simulink model "windEmulatorStep4"  (R2025b)
settings: Solver=ode4  StartTime=0.0  StopTime=inf  FixedStep=Ts  RelTol=1e-3
values from neighbouring files (symbols this model uses):
  A = 1.0    (= 1)    [initStep4.m]
  absEncoderCountsToRad = 1/2^20*2*pi    (= 5.99211245268e-06)    [initStep4.m]
  acs800CtrlStruct =     [windEmulatorBusDefs.mat]
  acs800DcBusVoltsScaling = 1    [initStep4.m]
  acs800FreqScaling = 1/100    (= 0.01)    [initStep4.m]
  acs800PowerScaling = Gen_PowerScaling    (= 14.9109)    [initStep4.m]
  acs800SignalStruct =     [windEmulatorBusDefs.mat]
  acs800SpeedNomEng = 1500    [initStep4.m]
  acs800SpeedNomFb = 20000    [initStep4.m]
  acs800SpeedScaling = 1500/20000    (= 0.075)    [initStep4.m]
  acs800TempScaling = 1/10    (= 0.1)    [initStep4.m]
  acs800TorqueNomEng = 100    [initStep4.m]
  acs800TorqueNomFb = 10000    [initStep4.m]
  acs800TorqueScaling = acs800TorqueRating/10000    (= 0.008035933)    [initStep4.m]
  acs880CtrlStruct =     [windEmulatorBusDefs.mat]
  acs880FreqScaling = 60/20000    (= 0.003)    [initStep4.m]
  acs880MotorCurrentScaling = 100/10000    (= 0.01)    [initStep4.m]
  acs880MotorVoltsScaling = 1    [initStep4.m]
  acs880PowerScaling = 100*hp2W/10000    (= 7.457)    [initStep4.m]
  acs880RatedTorque = 80.494    [initStep4.m]
  acs880RateLimFalling = -10000    [initStep4.m]
  acs880RateLimRising = 10000    [initStep4.m]
  acs880SetpointLimLower = -0.975*acs880RatedTorque    (= -78.48165)    [initStep4.m]
  acs880SetpointLimUpper = 0.975*acs880RatedTorque    (= 78.48165)    [initStep4.m]
  acs880SignalStruct =     [windEmulatorBusDefs.mat]
  acs880SpeedPILimLo = -0.975*acs880RatedTorque    (= -78.48165)    [initStep4.m]
  acs880SpeedPILimUp = 0.975*acs880RatedTorque    (= 78.48165)    [initStep4.m]
  acs880SpeedScaling = 2000/20000    (= 0.1)    [initStep4.m]
  acs880TorqueFieldbusScale = 10000    [initStep4.m]
  acs880TorqueScaling = acs880RatedTorque/acs880TorqueFieldbusScale    (= 0.0080494)    [initStep4.m]
  acs880TorqueSetpointScaling = 100    [initStep4.m]
  bar2pa = 1e5    (= 100000)    [initStep4.m]
  belowMinPGain = 1/200    (= 0.005)    [initStep4.m]
  ctrlModeTorque = logical(true)    [init.m]    (also in initStep1.m; initStep2.m; initStep3.m; initStep4.m)
  ctrlSignal1 = squeeze(hptoSignalsData.Values.ctrlSignal1.Data)    [postProcessingStep2.m]
  ctrlSignal2 = squeeze(hptoSignalsData.Values.ctrlSignal2.Data)    [postProcessingStep2.m]
  deadBandController = boolean(false)    [initStep4.m]
  deadbandTorqueSlewRate = 300    [initStep4.m]
  Dm_max = 40    [initStep4.m]
  EffMechMax = 0.93    [initStep4.m]
  EffMechMin = 0.79    [initStep4.m]
  excForce_N = squeeze(hptoCtrlData.Values.excForce_N.Data)    [postProcessingStep2.m]
  expCtrlStruct =     [windEmulatorBusDefs.mat]
  FactorEff = psi2pa*cc2m3*(1/rev2rad)    (= 0.00109733470463)    [initStep4.m]
  fromFileSpeedSlewRate = 250    [initStep4.m]
  fromFileTorqueSlewRate = 25    [initStep4.m]
  futekTorqueScale = -1/(2^31)*10/5*100    (= -9.31322574615e-08)    [initStep4.m]
  genMaxTorque = 0.8*ratedTorque    (= 64.3952)    [initStep3.m]    (also in initStep4.m = 78.48165)
  genTorqueCmd_Nm = squeeze(hptoSignalsData.Values.genTorqueCmd_Nm.Data)    [postProcessingStep2.m]
  hbmCtScale = 1/1.5    (= 0.666666666667)    [initStep4.m]
  hbmPowerStruct =     [windEmulatorBusDefs.mat]
  hptoCtrlStruct =     [windEmulatorBusDefs.mat]
  hptoSignalStruct =     [windEmulatorBusDefs.mat]
  invPowerStruct =     [windEmulatorBusDefs.mat]
  lpm2m3ps = 1/m3ps2lpm    (= 1.66666666667e-05)    [initStep4.m]
  minPressureRef_psi = 1000    [initStep4.m]
  minTorqueRef_Nm = (minPressureRef_psi*psi2pa)*(Dm_max*cc2m3*(1/rev2rad))    (= 43.8933881851)    [initStep4.m]
  motorSpeed_rpm = squeeze(acs880SignalsData.Values.motorSpeed_rpm.Data)    [postProcessingStep2.m]
  nPreDrop = 2900    [initStep4.m]
  nPreDropMin = 725    [initStep4.m]
  psi2bar = 1/bar2psi    (= 0.0689475729318)    [initStep4.m]
  radps2rpm = 60/(2*pi)    (= 9.54929658551)    [initStep2.m]    (also in initStep4.m)
  rpm2radps = 2*pi/60    (= 0.10471975512)    [initStep4.m]
  runCounter = squeeze(hptoCtrlData.Values.runCounter.Data)    [postProcessingStep2.m]
  shaftSignalStruct =     [windEmulatorBusDefs.mat]
  sidCtrlStruct =     [windEmulatorBusDefs.mat]
  sidDataCaseCounter = sidData.experimentData.count    [initStep4.m]
  sidDataSpeed_rpm = sidData.experimentData.wShaft_rpm    [initStep4.m]
  sidDataTorque_Nm = sidData.experimentData.torqueShaft_Nm    [initStep4.m]
  sidInfoStruct =     [windEmulatorBusDefs.mat]
  T = 4    [initStep4.m]
  targetOmega = 2000/60*2*pi    (= 209.439510239)    [initStep2.m]    (also in initStep3.m; initStep4.m)
  time = hptoCtrlData.Values.runCounter.Time    [postProcessingStep2.m]
  TorqueLoadMax = 75    [initStep4.m]
  Ts = 1/250    (= 0.004)    [initStep4.m]
undefined symbols (not defined in the file or in its folder): absEncoderCounts, absEncoderPosition_rad, absEncoderSpeed_rpm, absEncoderStatus1, absEncoderStatus2, absEncoderTurns, acs800Torque_Nm, acs800TorqueSetpoint_Nm, acs880SpeedSetpoint_rpm, acs880Torque_Nm, ctrlWord, dcBusVoltage_V, DiscIntNeverNeededParam, excShaftSpeed_rpm, excShaftTorque_Nm, expType, expTypeEnum, frequency_Hz, fromFileCaseCounter, genPumpFlow_lpm, genShaftSpeed_rpm, genSpeedActual, hmOutputShafTorque_Nm, motorCurrent_A, motorTorque_Nm, motorVoltage_V, pressure_bar, PressureControl, ramp, resetHilIntegrator, resetSidIntegrator, runHil, runSid, shaftPower_W, sidType, sidTypeEnum, SpeedControl, speedCtrlReset, speedRef_rpm, state, statusWord, stepCounter, temperature, torqueActual_Nm, TorqueInputControl, torqueSetpoint_Nm, torqueSetpoint_percent
libraries: slrealtimeethercatlib x118, fl_lib x26, nesl_utility x17, slrealtimeloglib x13, sh_lib x9, dspstat3 x5, simulink_extras x4, slpidlib x3, cstblocks x3, dspindex x3, simulink x2
(part 3 of 5)

== system windEmulatorStep4/fileAndUI/expCtrlSignalsUI ==
  expCtrlSignals : Inport  OutDataTypeStr=Bus: expCtrlBus
  Bus Selector : BusSelector  OutputSignals=expType,runHil,runSid,resetHilIntegrator,resetSidIntegrator,time,ramp,runCounter,stepCounter
  Constant : Constant  Value=true
  Terminator{,1..8} (9 alike) : Terminator
  expType : Bias  SaturateOnIntegerOverflow=off
  ramp : Gain
  resetHilIntegrator : Logic  IconShape=distinctive  AllPortsSameDT=off  OutDataTypeStr=boolean
  resetSidIntegrator : Logic  IconShape=distinctive  AllPortsSameDT=off  OutDataTypeStr=boolean
  runCounter : Bias  SaturateOnIntegerOverflow=off
  runHil : Logic  IconShape=distinctive  AllPortsSameDT=off  OutDataTypeStr=boolean
  runSid : Logic  IconShape=distinctive  AllPortsSameDT=off  OutDataTypeStr=boolean
  stepCounter : Bias  SaturateOnIntegerOverflow=off
  time : Gain
  wires:
  expCtrlSignals/1 -> Bus Selector/1
  Bus Selector/1 -> expType/1  "<expType>"
  expType/1 -> Terminator/1
  Bus Selector/2 -> runHil/2  "<runHil>"
  Constant/1 -> resetSidIntegrator/1, resetHilIntegrator/1, runSid/1, runHil/1
  runHil/1 -> Terminator1/1
  Bus Selector/3 -> runSid/2  "<runSid>"
  runSid/1 -> Terminator2/1
  Bus Selector/4 -> resetHilIntegrator/2  "<resetHilIntegrator>"
  resetHilIntegrator/1 -> Terminator3/1
  Bus Selector/5 -> resetSidIntegrator/2  "<resetSidIntegrator>"
  resetSidIntegrator/1 -> Terminator4/1
  Bus Selector/8 -> runCounter/1  "<runCounter>"
  runCounter/1 -> Terminator5/1
  Bus Selector/6 -> time/1  "<time>"
  time/1 -> Terminator6/1
  Bus Selector/7 -> ramp/1  "<ramp>"
  ramp/1 -> Terminator7/1
  Bus Selector/9 -> stepCounter/1  "<stepCounter>"
  stepCounter/1 -> Terminator8/1

== system windEmulatorStep4/fileAndUI/hptoCtrlSignalsUI ==
  hptoCtrlSignals : Inport  OutDataTypeStr=Bus: hptoCtrlBus
  Bus Selector : BusSelector  OutputSignals=speedRef_rpm,excForce_N,genSpeedActual,speedCtrlReset
  Terminator{,1,4,6} (4 alike) : Terminator
  excForce_N : Gain
  genSpeedActual : Gain
  speedCtrlReset : Gain
  speedRef_rpm : Gain
  wires:
  hptoCtrlSignals/1 -> Bus Selector/1
  Bus Selector/1 -> speedRef_rpm/1  "<speedRef_rpm>"
  speedRef_rpm/1 -> Terminator/1
  Bus Selector/2 -> excForce_N/1  "<excForce_N>"
  excForce_N/1 -> Terminator1/1
  Bus Selector/3 -> genSpeedActual/1  "<genSpeedActual>"
  genSpeedActual/1 -> Terminator4/1
  Bus Selector/4 -> speedCtrlReset/1  "<speedCtrlReset>"
  speedCtrlReset/1 -> Terminator6/1

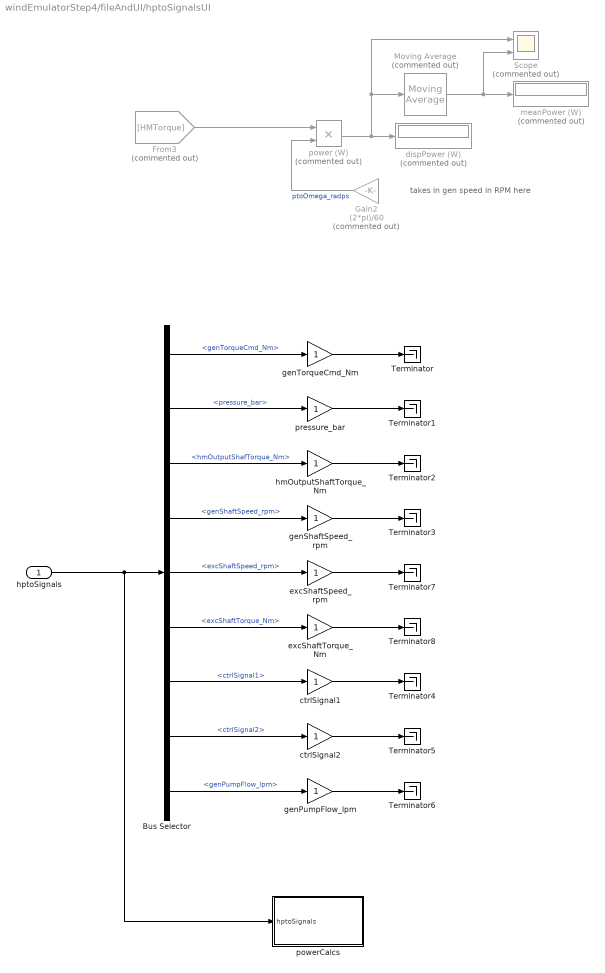
== system windEmulatorStep4/fileAndUI/hptoSignalsUI ==
  note: takes in gen speed in RPM here
  hptoSignals : Inport  OutDataTypeStr=Bus: hptoSignalBus
  Bus Selector : BusSelector  OutputSignals=genTorqueCmd_Nm,pressure_bar,hmOutputShafTorque_Nm,genShaftSpeed_rpm,excShaftSpeed_rpm,excShaftTorque_Nm,ctrlSignal1,ctrlSignal2,genPumpFlow_lpm
  From3 : From  Commented=on  GotoTag=HMTorque
  Gain2 : Gain  Commented=on  Gain=(2*pi)/60
  Moving Average : dspstat3/Moving Average  Commented=on  Method=Sliding window  ForgettingFactorPort=off  SpecifyWindowLength=on  WindowLength=20*500  OverlapLength=9999  AllowArbitraryInputLength=off  ForgettingFactor=0.9  SimulateUsing=Code generation
  Scope : Scope  Commented=on  NumInputPorts=2
      settings: ActiveDisplayYMinimum=-287.86927  ActiveDisplayYMaximum=31.98547
  Terminator{,1..8} (9 alike) : Terminator
  ctrlSignal1 : Gain
  ctrlSignal2 : Gain
  dispPower (W) : Display  Commented=on
  excShaftSpeed_rpm : Gain
  excShaftTorque_Nm : Gain
  genPumpFlow_lpm : Gain
  genShaftSpeed_rpm : Gain
  genTorqueCmd_Nm : Gain
  hmOutputShaftTorque_Nm : Gain
  meanPower (W) : Display  Commented=on
  power (W) : Product  Commented=on
  powerCalcs : Subsystem
  pressure_bar : Gain
  wires:
  hptoSignals/1 -> powerCalcs/1(hptoSignals), Bus Selector/1
  Bus Selector/1 -> genTorqueCmd_Nm/1  "<genTorqueCmd_Nm>"
  genTorqueCmd_Nm/1 -> Terminator/1
  Bus Selector/2 -> pressure_bar/1  "<pressure_bar>"
  pressure_bar/1 -> Terminator1/1
  Bus Selector/3 -> hmOutputShaftTorque_Nm/1  "<hmOutputShafTorque_Nm>"
  hmOutputShaftTorque_Nm/1 -> Terminator2/1
  Bus Selector/4 -> genShaftSpeed_rpm/1  "<genShaftSpeed_rpm>"
  genShaftSpeed_rpm/1 -> Terminator3/1
  Bus Selector/7 -> ctrlSignal1/1  "<ctrlSignal1>"
  ctrlSignal1/1 -> Terminator4/1
  Bus Selector/8 -> ctrlSignal2/1  "<ctrlSignal2>"
  ctrlSignal2/1 -> Terminator5/1
  Bus Selector/9 -> genPumpFlow_lpm/1  "<genPumpFlow_lpm>"
  genPumpFlow_lpm/1 -> Terminator6/1
  From3/1 -> power (W)/1
  power (W)/1 -> Scope/1, Moving Average/1, dispPower (W)/1
  Moving Average/1 -> Scope/2, meanPower (W)/1
  Gain2/1 -> power (W)/2  "ptoOmega_radps"
  Bus Selector/5 -> excShaftSpeed_rpm/1  "<excShaftSpeed_rpm>"
  excShaftSpeed_rpm/1 -> Terminator7/1
  Bus Selector/6 -> excShaftTorque_Nm/1  "<excShaftTorque_Nm>"
  excShaftTorque_Nm/1 -> Terminator8/1

== system windEmulatorStep4/fileAndUI/shaftSignalsUI ==
  shaftSignals : Inport  OutDataTypeStr=Bus: shaftSignalBus
  Bus Selector : BusSelector  OutputSignals=torqueActual_Nm,absEncoderCounts,absEncoderTurns,absEncoderPosition_rad,absEncoderSpeed_rpm,absEncoderStatus1,absEncoderStatus2
  Terminator{,1..6} (7 alike) : Terminator
  absEncoderCounts : Bias  SaturateOnIntegerOverflow=off
  absEncoderPosition_rad : Gain
  absEncoderSpeed_rpm : Gain
  absEncoderStatus1 : Bias  SaturateOnIntegerOverflow=off
  absEncoderStatus2 : Bias  SaturateOnIntegerOverflow=off
  absEncoderTurns : Bias  SaturateOnIntegerOverflow=off
  torqueActual_Nm : Gain
  wires:
  shaftSignals/1 -> Bus Selector/1
  Bus Selector/1 -> torqueActual_Nm/1  "<torqueActual_Nm>"
  absEncoderPosition_rad/1 -> Terminator/1
  torqueActual_Nm/1 -> Terminator1/1
  absEncoderStatus1/1 -> Terminator2/1
  Bus Selector/2 -> absEncoderCounts/1  "<absEncoderCounts>"
  Bus Selector/4 -> absEncoderPosition_rad/1  "<absEncoderPosition_rad>"
  absEncoderCounts/1 -> Terminator3/1
  Bus Selector/5 -> absEncoderSpeed_rpm/1  "<absEncoderSpeed_rpm>"
  absEncoderSpeed_rpm/1 -> Terminator4/1
  Bus Selector/6 -> absEncoderStatus1/1  "<absEncoderStatus1>"
  Bus Selector/7 -> absEncoderStatus2/1  "<absEncoderStatus2>"
  absEncoderStatus2/1 -> Terminator5/1
  Bus Selector/3 -> absEncoderTurns/1  "<absEncoderTurns>"
  absEncoderTurns/1 -> Terminator6/1

== system windEmulatorStep4/hptoSim/hptoModel ==
  speedReference : Inport
  genSpeedActual_rpm : Inport  Port=2
  excForce_N : Inport  Port=3
  speedControllerReset : Inport  Port=4
  Constant1 : Constant  Value=minPressureRef_psi
  ControlAlgorithm : Subsystem
      settings: PortSchema="{\"entries\":[{\"content\":{\"sides\":[{\"content\":{\"connectorIds\":[\"In1\",\"In2\",\"In3\"]},\"type\":\"ConnectorPlacement.EquallySpacedRectSide\",\"uuid\":\"67adeffe-a398-49a8-b4a5-c43e48a316d9\"},{\"content\":{\"connectorIds\":[\"Out1\",\"Out2\",\"Out3\"],\"side\":\"RIGHT\"},\"type\":\"ConnectorPlacement.EquallySpacedRectSide\",\"uuid\":\"a2794d83-d293-4f11-b47e-435bf1d282f7\"},{\"content\":{\"connectorIds\":[],\"side\":\"TOP\"},\"type\":\"ConnectorPlacement.EquallySpacedRectSide\",\"uuid\":\"bb9f1178-f133-4eb3-bddb-bcb3a714b020\"},{\"content\":{\"connectorIds\":[\"In4\"],\"side\":\"BOTTOM\"},\"type\":\"ConnectorPlacement.EquallySpacedRectSide\",\"uuid\":\"388d2827-2454-4d01-b75f-f317c9ccd7ab\"}]},\"type\":\"ConnectorPlacement.EquallySpacedConnector\",\"uuid\":\"ef44af23-246a-43fe-a184-a2d38abebfbf\"}],\"packageUris\":[\"http://schema.mathworks.com/mf0/Connector/R2020b\"],\"version\":\"1.0\"}"
  HPTO : Subsystem
      settings: PortSchema="{\"entries\":[{\"content\":{\"sides\":[{\"content\":{\"connectorIds\":[\"In1\",\"In2\"]},\"type\":\"ConnectorPlacement.EquallySpacedRectSide\",\"uuid\":\"8fa4c7ba-45c7-41ba-9bcd-58cbee0318ba\"},{\"content\":{\"connectorIds\":[\"Out1\",\"Out2\",\"Out3\",\"Out4\",\"Out5\",\"Out6\",\"Out7\"],\"side\":\"RIGHT\"},\"type\":\"ConnectorPlacement.EquallySpacedRectSide\",\"uuid\":\"a23e9dd6-a871-47ae-a82a-10ea55782587\"},{\"content\":{\"connectorIds\":[\"In3\",\"In4\"],\"side\":\"TOP\"},\"type\":\"ConnectorPlacement.EquallySpacedRectSide\",\"uuid\":\"238aec0c-a47f-4ecc-bf69-7ee7f3fea80c\"}]},\"type\":\"ConnectorPlacement.EquallySpacedConnector\",\"uuid\":\"c89831dd-0ad8-4547-8547-63f84e5efa4b\"}],\"packageUris\":[\"http://schema.mathworks.com/mf0/Connector/R2020b\"],\"version\":\"1.0\"}"
  genTorqueCmd_Nm : Outport
  pressure_psi : Outport  Port=2
  hmOutputShaftTorque_Nm : Outport  Port=3
  genShaftSpeed_rpm : Outport  Port=4
  excShaftSpeed_rpm : Outport  Port=5
  excShaftTorque_Nm : Outport  Port=6
  controlSignal1 : Outport  Port=7
  controlSignal2 : Outport  Port=8
  genPumpFlow_lpm : Outport  Port=9
  wires:
  HPTO/1(SystemOutputs) -> ControlAlgorithm/4(ActualSignals)
  ControlAlgorithm/1(ControlSignal1) -> HPTO/1(ControlSignal1), controlSignal1/1  "ControlSignal1"
  Constant1/1 -> ControlAlgorithm/1(minPressureRef)  "minPressureRef"
  ControlAlgorithm/2(ControlSignal2) -> HPTO/2(ControlSignal2), controlSignal2/1  "ControlSignal2"
  excForce_N/1 -> HPTO/3(Fexc)
  genSpeedActual_rpm/1 -> HPTO/4(genSpeedActual_rpm)
  HPTO/2(Pressure) -> pressure_psi/1
  ControlAlgorithm/3(ControlTorqueLoad) -> genTorqueCmd_Nm/1  "ControlTorqueLoad"
  speedControllerReset/1 -> ControlAlgorithm/3(SpeedControllerReset)
  speedReference/1 -> ControlAlgorithm/2(ShaftSpeedRef)
  HPTO/3(hmOutputShaftTorque) -> hmOutputShaftTorque_Nm/1
  HPTO/4(genShaftSpeed_rpm) -> genShaftSpeed_rpm/1
  HPTO/7(genPumpFlow_lpm) -> genPumpFlow_lpm/1
  HPTO/5(excShaftSpeed_rpm) -> excShaftSpeed_rpm/1
  HPTO/6(excShaftTorque_Nm) -> excShaftTorque_Nm/1

== system windEmulatorStep4/readShaftSignals/countsToRads ==
  note: This logic detects a jump in encoder position, and adds or removes a turn
  note: The encoder has a resolution of 20 bits / rev. If we detect a jump of more than 2^19, we add or remove 1 turn
  rawCounts : Inport  OutDataTypeStr=uint32
  Abs : Abs  OutDataTypeStr=int32  SaturateOnIntegerOverflow=off
  Add : Sum  Inputs=+-
  Add1 : Sum  OutDataTypeStr=int32
  Add2 : Sum
  Cast To Double : DataTypeConversion  OutDataTypeStr=int32  SaturateOnIntegerOverflow=off  RndMeth=Floor
  Cast To Double1 : DataTypeConversion  OutDataTypeStr=double  SaturateOnIntegerOverflow=off  RndMeth=Floor
  Cast To Double3 : DataTypeConversion  OutDataTypeStr=double  SaturateOnIntegerOverflow=off  RndMeth=Floor
  Constant : Constant  Value=2^19  OutDataTypeStr=int32
  Constant1 : Constant  Value=0  OutDataTypeStr=int32
  Gain : Gain  Gain=2*pi
  Relational Operator : RelationalOperator  OutDataTypeStr=boolean  RndMeth=Simplest  InputSameDT=off
  Sign : Signum
  Switch : Switch  Criteria=u2 > Threshold  OutDataTypeStr=int32  SaturateOnIntegerOverflow=off  InputSameDT=off
  encoderCountsToRad : Gain  Gain=absEncoderCountsToRad
  lastRawCounts : Memory
  lastTurn : Memory
  turns : Outport  OutDataTypeStr=int32
  pos_rad : Outport  Port=2
  wires:
  Cast To Double3/1 -> encoderCountsToRad/1
  Constant/1 -> Relational Operator/2
  Relational Operator/1 -> Switch/2
  Constant1/1 -> Switch/3
  rawCounts/1 -> Cast To Double/1
  Add/1 -> Sign/1, Abs/1
  Add1/1 -> turns/1, lastTurn/1, Cast To Double1/1
  encoderCountsToRad/1 -> Add2/1
  Gain/1 -> Add2/2
  Add2/1 -> pos_rad/1
  Abs/1 -> Relational Operator/1
  Sign/1 -> Switch/1
  lastTurn/1 -> Add1/2
  Cast To Double1/1 -> Gain/1
  Cast To Double/1 -> Add/2, lastRawCounts/1, Cast To Double3/1
  Switch/1 -> Add1/1
  lastRawCounts/1 -> Add/1

== system windEmulatorStep4/sidCtrl/setpointGenerator ==
  note: Hold ramp at zero if not running SID
  expCtrl : Inport  OutDataTypeStr=Bus: expCtrlBus
  inportSpeed_rpm : Inport  Port=2
  inportTorque_Nm : Inport  Port=3
  inportCaseCounter : Inport  Port=4
  Bus Assignment : BusAssignment  AssignedSignals=acs800TorqueSetpoint_Nm,acs880SpeedSetpoint_rpm,sidType,fromFileCaseCounter
  Bus Selector : BusSelector  OutputSignals=ramp,runSid
  Cast To uint32 : DataTypeConversion  OutDataTypeStr=uint32  SaturateOnIntegerOverflow=off  RndMeth=Floor
  Constant : Constant  Value=sidInfoStruct  OutDataTypeStr=Bus: sidInfoBus
  Constant1 : Constant  Value=0
  Constant3 : Constant  Value=0
  Multiport Switch : MultiPortSwitch  DataPortOrder=Specify indices  DataPortIndices={sidTypeEnum.off,sidTypeEnum.manual,sidTypeEnum.fromFile}  DataPortForDefault=Additional data port  SaturateOnIntegerOverflow=off  InputSameDT=off
  Multiport Switch1 : MultiPortSwitch  DataPortOrder=Specify indices  DataPortIndices={sidTypeEnum.off,sidTypeEnum.manual,sidTypeEnum.fromFile}  DataPortForDefault=Additional data port  SaturateOnIntegerOverflow=off  InputSameDT=off
  Product : Product
  Product1 : Product
  Switch : Switch  Criteria=u2 > Threshold  SaturateOnIntegerOverflow=off  InputSameDT=off
  fromFile : Subsystem
  manualSpeedSetpoint_rpm : Constant  Value=0
  manualTorqueSetpoint_Nm : Constant  Value=0
  sidType : Constant  Value=sidTypeEnum.off  OutDataTypeStr=Enum: sidTypeEnum
  acs800TorqueSetpoint_Nm : Outport
  acs880SpeedSetpoint_rpm : Outport  Port=2
  sidInfoSignals : Outport  Port=3  OutDataTypeStr=Bus: sidInfoBus
  wires:
  Constant3/1 -> Multiport Switch1/5, Multiport Switch1/2, Multiport Switch/5, Multiport Switch/2
  manualTorqueSetpoint_Nm/1 -> Multiport Switch/3
  manualSpeedSetpoint_rpm/1 -> Multiport Switch1/3
  expCtrl/1 -> fromFile/2(expCtrl), Bus Selector/1
  Bus Selector/2 -> Switch/2  "<runSid>"
  Bus Selector/1 -> Switch/1  "<ramp>"
  Constant1/1 -> Switch/3
  Multiport Switch/1 -> Product/2
  Switch/1 -> Product/1, Product1/1  "rampValue"
  Product/1 -> acs800TorqueSetpoint_Nm/1, Bus Assignment/2
  Multiport Switch1/1 -> Product1/2
  Product1/1 -> Bus Assignment/3, acs880SpeedSetpoint_rpm/1
  fromFile/1(torqueSetpoint_rpm) -> Multiport Switch/4
  fromFile/2(speedSetpoint_rpm) -> Multiport Switch1/4
  sidType/1 -> Cast To uint32/1, fromFile/1(sidType), Multiport Switch1/1, Multiport Switch/1
  Constant/1 -> Bus Assignment/1
  fromFile/3(caseCounter) -> Bus Assignment/5
  Bus Assignment/1 -> sidInfoSignals/1
  Cast To uint32/1 -> Bus Assignment/4
  inportSpeed_rpm/1 -> fromFile/3(inportSpeed_rpm)
  inportTorque_Nm/1 -> fromFile/4(inportTorque_Nm)
  inportCaseCounter/1 -> fromFile/5(inportCaseCounter)

== system windEmulatorStep4/writeAcs800Pdos/ACS800ConvertREF1 ==
  Eng : Inport
  Constant EngineeringValue : Constant  Value=EngineeringValue
  Constant FieldbusValue : Constant  Value=FieldbusValue
  Product : Product  Inputs=**/
  Fb : Outport
  wires:
  Constant EngineeringValue/1 -> Product/3
  Constant FieldbusValue/1 -> Product/2
  Eng/1 -> Product/1
  Product/1 -> Fb/1

== system windEmulatorStep4/writeAcs800Pdos/ACS800ConvertREF2 ==
  Eng : Inport
  Constant EngineeringValue : Constant  Value=EngineeringValue
  Constant FieldbusValue : Constant  Value=FieldbusValue
  Product : Product  Inputs=**/
  Fb : Outport
  wires:
  Constant EngineeringValue/1 -> Product/3
  Constant FieldbusValue/1 -> Product/2
  Eng/1 -> Product/1
  Product/1 -> Fb/1

== system windEmulatorStep4/writeAcs880Pdos/ACS880ConvertREF2 ==
  Eng : Inport
  Constant EngineeringValue : Constant  Value=EngineeringValue
  Constant FieldbusValue : Constant  Value=FieldbusValue
  Product : Product  Inputs=**/
  Fb : Outport
  wires:
  Product/1 -> Fb/1
  Eng/1 -> Product/1
  Constant FieldbusValue/1 -> Product/2
  Constant EngineeringValue/1 -> Product/3

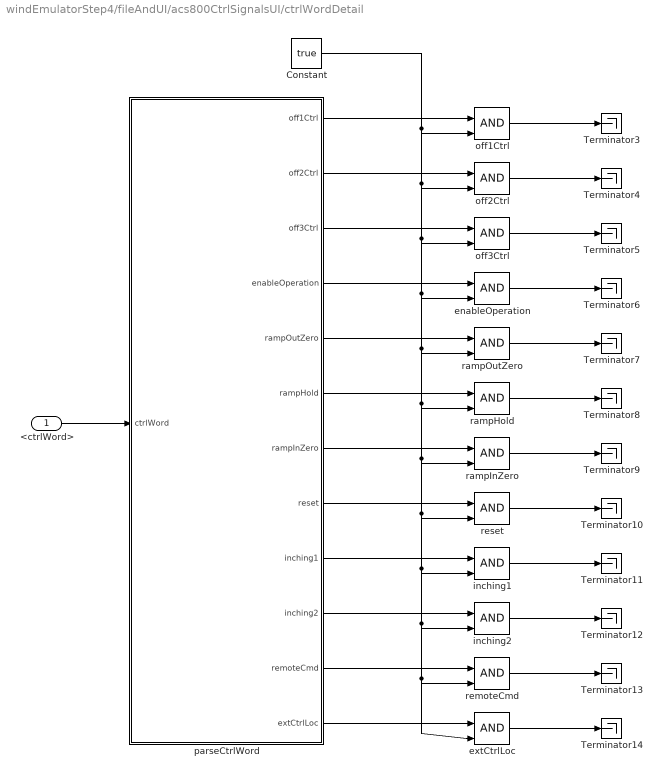
== system windEmulatorStep4/fileAndUI/acs800CtrlSignalsUI/ctrlWordDetail ==
  <ctrlWord> : Inport
  Constant : Constant  Value=true  OutDataTypeStr=boolean
  Terminator{3..14} (12 alike) : Terminator
  enableOperation : Logic  IconShape=distinctive  AllPortsSameDT=off  OutDataTypeStr=boolean
  extCtrlLoc : Logic  IconShape=distinctive  AllPortsSameDT=off  OutDataTypeStr=boolean
  inching1 : Logic  IconShape=distinctive  AllPortsSameDT=off  OutDataTypeStr=boolean
  inching2 : Logic  IconShape=distinctive  AllPortsSameDT=off  OutDataTypeStr=boolean
  off1Ctrl : Logic  IconShape=distinctive  AllPortsSameDT=off  OutDataTypeStr=boolean
  off2Ctrl : Logic  IconShape=distinctive  AllPortsSameDT=off  OutDataTypeStr=boolean
  off3Ctrl : Logic  IconShape=distinctive  AllPortsSameDT=off  OutDataTypeStr=boolean
  parseCtrlWord : MATLAB Function  TreatAsAtomicUnit=on
  rampHold : Logic  IconShape=distinctive  AllPortsSameDT=off  OutDataTypeStr=boolean
  rampInZero : Logic  IconShape=distinctive  AllPortsSameDT=off  OutDataTypeStr=boolean
  rampOutZero : Logic  IconShape=distinctive  AllPortsSameDT=off  OutDataTypeStr=boolean
  remoteCmd : Logic  IconShape=distinctive  AllPortsSameDT=off  OutDataTypeStr=boolean
  reset : Logic  IconShape=distinctive  AllPortsSameDT=off  OutDataTypeStr=boolean
  wires:
  reset/1 -> Terminator10/1
  Constant/1 -> off3Ctrl/2, rampInZero/2, extCtrlLoc/2, remoteCmd/2, inching2/2, inching1/2, reset/2, rampHold/2, rampOutZero/2, enableOperation/2, off2Ctrl/2, off1Ctrl/2
  parseCtrlWord/11(remoteCmd) -> remoteCmd/1
  enableOperation/1 -> Terminator6/1
  inching2/1 -> Terminator12/1
  off2Ctrl/1 -> Terminator4/1
  <ctrlWord>/1 -> parseCtrlWord/1(ctrlWord)
  parseCtrlWord/7(rampInZero) -> rampInZero/1
  off3Ctrl/1 -> Terminator5/1
  parseCtrlWord/8(reset) -> reset/1
  rampHold/1 -> Terminator8/1
  parseCtrlWord/2(off2Ctrl) -> off2Ctrl/1
  off1Ctrl/1 -> Terminator3/1
  rampOutZero/1 -> Terminator7/1
  parseCtrlWord/6(rampHold) -> rampHold/1
  parseCtrlWord/9(inching1) -> inching1/1
  rampInZero/1 -> Terminator9/1
  parseCtrlWord/5(rampOutZero) -> rampOutZero/1
  parseCtrlWord/3(off3Ctrl) -> off3Ctrl/1
  parseCtrlWord/12(extCtrlLoc) -> extCtrlLoc/1
  remoteCmd/1 -> Terminator13/1
  extCtrlLoc/1 -> Terminator14/1
  parseCtrlWord/1(off1Ctrl) -> off1Ctrl/1
  inching1/1 -> Terminator11/1
  parseCtrlWord/4(enableOperation) -> enableOperation/1
  parseCtrlWord/10(inching2) -> inching2/1

== system windEmulatorStep4/fileAndUI/acs800SignalsUI/powerCals ==
  acs800Signals : Inport  OutDataTypeStr=Bus: acs800SignalBus
  Bus Selector : BusSelector  OutputSignals=motorSpeed_rpm,motorTorque_Nm
  Moving Average : dspstat3/Moving Average  Method=Sliding window  ForgettingFactorPort=off  SpecifyWindowLength=on  WindowLength=movingAverageLength  OverlapLength=2499  AllowArbitraryInputLength=off  ForgettingFactor=0.9  SimulateUsing=Code generation
  Product : Product
  Terminator : Terminator
  Terminator1 : Terminator
  "rpm -> rad/s" : Gain  Gain=rpm2radps
  shaftPowerAverage_W : Gain
  shaftPower_W : Gain
  wires:
  acs800Signals/1 -> Bus Selector/1
  Bus Selector/1 -> "rpm -> rad/s"/1  "<motorSpeed_rpm>"
  "rpm -> rad/s"/1 -> Product/1
  Bus Selector/2 -> Product/2  "<motorTorque_Nm>"
  Product/1 -> Moving Average/1, shaftPower_W/1
  shaftPower_W/1 -> Terminator/1
  Moving Average/1 -> shaftPowerAverage_W/1
  shaftPowerAverage_W/1 -> Terminator1/1

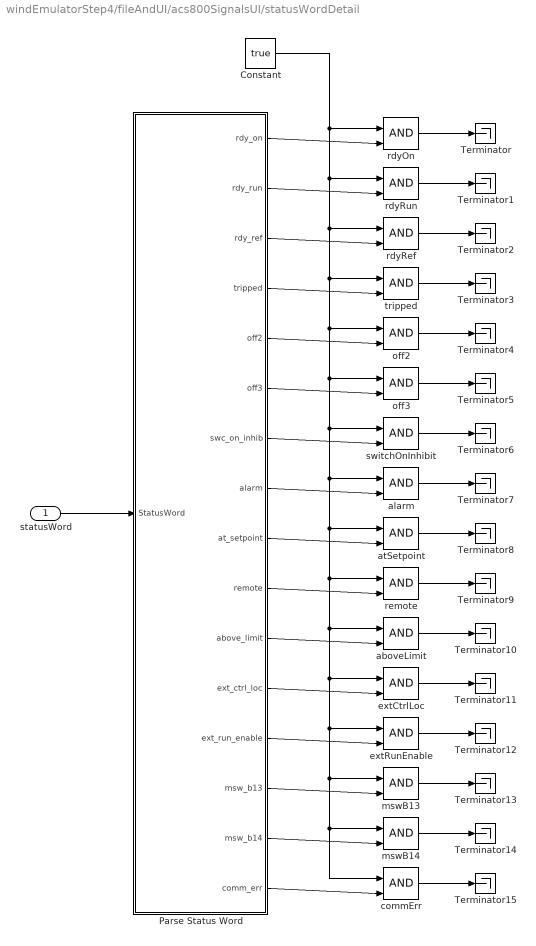
== system windEmulatorStep4/fileAndUI/acs800SignalsUI/statusWordDetail ==
  statusWord : Inport
  Constant : Constant  Value=true  OutDataTypeStr=boolean
  Parse Status Word : MATLAB Function  TreatAsAtomicUnit=on
  Terminator{,1..15} (16 alike) : Terminator
  aboveLimit : Logic  IconShape=distinctive  AllPortsSameDT=off  OutDataTypeStr=boolean
  alarm : Logic  IconShape=distinctive  AllPortsSameDT=off  OutDataTypeStr=boolean
  atSetpoint : Logic  IconShape=distinctive  AllPortsSameDT=off  OutDataTypeStr=boolean
  commErr : Logic  IconShape=distinctive  AllPortsSameDT=off  OutDataTypeStr=boolean
  extCtrlLoc : Logic  IconShape=distinctive  AllPortsSameDT=off  OutDataTypeStr=boolean
  extRunEnable : Logic  IconShape=distinctive  AllPortsSameDT=off  OutDataTypeStr=boolean
  mswB13 : Logic  IconShape=distinctive  AllPortsSameDT=off  OutDataTypeStr=boolean
  mswB14 : Logic  IconShape=distinctive  AllPortsSameDT=off  OutDataTypeStr=boolean
  off2 : Logic  IconShape=distinctive  AllPortsSameDT=off  OutDataTypeStr=boolean
  off3 : Logic  IconShape=distinctive  AllPortsSameDT=off  OutDataTypeStr=boolean
  rdyOn : Logic  IconShape=distinctive  AllPortsSameDT=off  OutDataTypeStr=boolean
  rdyRef : Logic  IconShape=distinctive  AllPortsSameDT=off  OutDataTypeStr=boolean
  rdyRun : Logic  IconShape=distinctive  AllPortsSameDT=off  OutDataTypeStr=boolean
  remote : Logic  IconShape=distinctive  AllPortsSameDT=off  OutDataTypeStr=boolean
  switchOnInhibit : Logic  IconShape=distinctive  AllPortsSameDT=off  OutDataTypeStr=boolean
  tripped : Logic  IconShape=distinctive  AllPortsSameDT=off  OutDataTypeStr=boolean
  wires:
  statusWord/1 -> Parse Status Word/1(StatusWord)
  Parse Status Word/1(rdy_on) -> rdyOn/2
  Constant/1 -> mswB13/1, commErr/1, mswB14/1, extRunEnable/1, extCtrlLoc/1, aboveLimit/1, remote/1, atSetpoint/1, alarm/1, switchOnInhibit/1, off3/1, off2/1, tripped/1, rdyRef/1, rdyRun/1, rdyOn/1
  rdyOn/1 -> Terminator/1
  rdyRun/1 -> Terminator1/1
  Parse Status Word/2(rdy_run) -> rdyRun/2
  rdyRef/1 -> Terminator2/1
  tripped/1 -> Terminator3/1
  Parse Status Word/4(tripped) -> tripped/2
  Parse Status Word/5(off2) -> off2/2
  off2/1 -> Terminator4/1
  off3/1 -> Terminator5/1
  Parse Status Word/6(off3) -> off3/2
  Parse Status Word/7(swc_on_inhib) -> switchOnInhibit/2
  switchOnInhibit/1 -> Terminator6/1
  alarm/1 -> Terminator7/1
  Parse Status Word/8(alarm) -> alarm/2
  Parse Status Word/9(at_setpoint) -> atSetpoint/2
  atSetpoint/1 -> Terminator8/1
  remote/1 -> Terminator9/1
  Parse Status Word/10(remote) -> remote/2
  Parse Status Word/11(above_limit) -> aboveLimit/2
  aboveLimit/1 -> Terminator10/1
  extCtrlLoc/1 -> Terminator11/1
  Parse Status Word/12(ext_ctrl_loc) -> extCtrlLoc/2
  Parse Status Word/13(ext_run_enable) -> extRunEnable/2
  extRunEnable/1 -> Terminator12/1
  mswB13/1 -> Terminator13/1
  Parse Status Word/14(msw_b13) -> mswB13/2
  Parse Status Word/15(msw_b14) -> mswB14/2
  mswB14/1 -> Terminator14/1
  commErr/1 -> Terminator15/1
  Parse Status Word/16(comm_err) -> commErr/2
  Parse Status Word/3(rdy_ref) -> rdyRef/2

== system windEmulatorStep4/fileAndUI/acs880CtrlSignalsUI/ctrlWordDetail ==
  <ctrlWord> : Inport
  Constant : Constant  Value=true  OutDataTypeStr=boolean
  Terminator{3..14} (12 alike) : Terminator
  enableOperation : Logic  IconShape=distinctive  AllPortsSameDT=off  OutDataTypeStr=boolean
  extCtrlLoc : Logic  IconShape=distinctive  AllPortsSameDT=off  OutDataTypeStr=boolean
  inching1 : Logic  IconShape=distinctive  AllPortsSameDT=off  OutDataTypeStr=boolean
  inching2 : Logic  IconShape=distinctive  AllPortsSameDT=off  OutDataTypeStr=boolean
  off1Ctrl : Logic  IconShape=distinctive  AllPortsSameDT=off  OutDataTypeStr=boolean
  off2Ctrl : Logic  IconShape=distinctive  AllPortsSameDT=off  OutDataTypeStr=boolean
  off3Ctrl : Logic  IconShape=distinctive  AllPortsSameDT=off  OutDataTypeStr=boolean
  parseCtrlWord : MATLAB Function  TreatAsAtomicUnit=on
  rampHold : Logic  IconShape=distinctive  AllPortsSameDT=off  OutDataTypeStr=boolean
  rampInZero : Logic  IconShape=distinctive  AllPortsSameDT=off  OutDataTypeStr=boolean
  rampOutZero : Logic  IconShape=distinctive  AllPortsSameDT=off  OutDataTypeStr=boolean
  remoteCmd : Logic  IconShape=distinctive  AllPortsSameDT=off  OutDataTypeStr=boolean
  reset : Logic  IconShape=distinctive  AllPortsSameDT=off  OutDataTypeStr=boolean
  wires:
  reset/1 -> Terminator10/1
  Constant/1 -> off3Ctrl/2, rampInZero/2, extCtrlLoc/2, remoteCmd/2, inching2/2, inching1/2, reset/2, rampHold/2, rampOutZero/2, enableOperation/2, off2Ctrl/2, off1Ctrl/2
  parseCtrlWord/11(remoteCmd) -> remoteCmd/1
  enableOperation/1 -> Terminator6/1
  inching2/1 -> Terminator12/1
  off2Ctrl/1 -> Terminator4/1
  <ctrlWord>/1 -> parseCtrlWord/1(ctrlWord)
  parseCtrlWord/7(rampInZero) -> rampInZero/1
  off3Ctrl/1 -> Terminator5/1
  parseCtrlWord/8(reset) -> reset/1
  rampHold/1 -> Terminator8/1
  parseCtrlWord/2(off2Ctrl) -> off2Ctrl/1
  off1Ctrl/1 -> Terminator3/1
  rampOutZero/1 -> Terminator7/1
  parseCtrlWord/6(rampHold) -> rampHold/1
  parseCtrlWord/9(inching1) -> inching1/1
  rampInZero/1 -> Terminator9/1
  parseCtrlWord/5(rampOutZero) -> rampOutZero/1
  parseCtrlWord/3(off3Ctrl) -> off3Ctrl/1
  parseCtrlWord/12(extCtrlLoc) -> extCtrlLoc/1
  remoteCmd/1 -> Terminator13/1
  extCtrlLoc/1 -> Terminator14/1
  parseCtrlWord/1(off1Ctrl) -> off1Ctrl/1
  inching1/1 -> Terminator11/1
  parseCtrlWord/4(enableOperation) -> enableOperation/1
  parseCtrlWord/10(inching2) -> inching2/1

== system windEmulatorStep4/fileAndUI/acs880SignalsUI/powerCals ==
  acs880Signals : Inport  OutDataTypeStr=Bus: acs880SignalBus
  Bus Selector : BusSelector  OutputSignals=motorSpeed_rpm,motorTorque_Nm
  Moving Average : dspstat3/Moving Average  Method=Sliding window  ForgettingFactorPort=off  SpecifyWindowLength=on  WindowLength=movingAverageLength  OverlapLength=2499  AllowArbitraryInputLength=off  ForgettingFactor=0.9  SimulateUsing=Code generation
  Product : Product
  Terminator : Terminator
  Terminator1 : Terminator
  "rpm -> rad/s" : Gain  Gain=rpm2radps
  shaftPowerAverage_W : Gain
  shaftPower_W : Gain
  wires:
  Bus Selector/1 -> "rpm -> rad/s"/1  "<motorSpeed_rpm>"
  "rpm -> rad/s"/1 -> Product/1
  Bus Selector/2 -> Product/2  "<motorTorque_Nm>"
  Product/1 -> Moving Average/1, shaftPower_W/1
  shaftPower_W/1 -> Terminator/1
  acs880Signals/1 -> Bus Selector/1
  shaftPowerAverage_W/1 -> Terminator1/1
  Moving Average/1 -> shaftPowerAverage_W/1

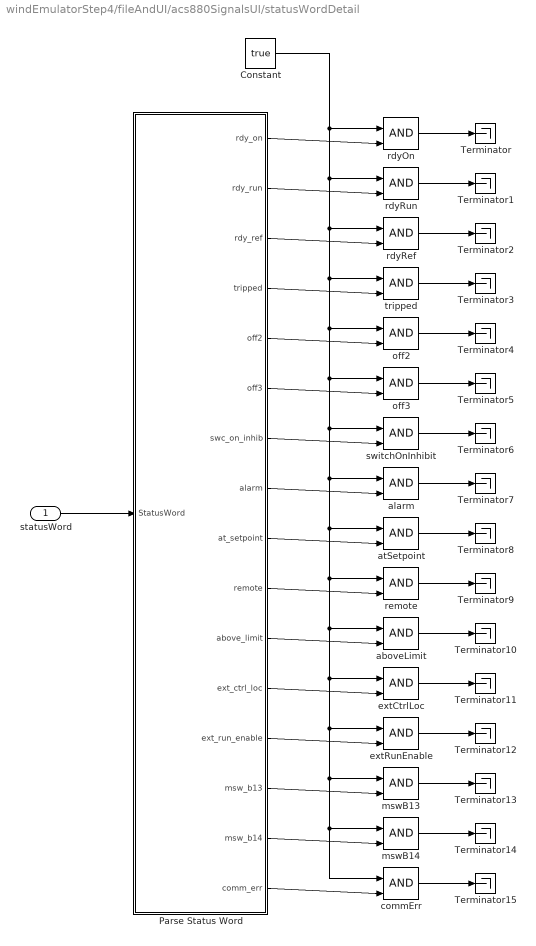
== system windEmulatorStep4/fileAndUI/acs880SignalsUI/statusWordDetail ==
  statusWord : Inport
  Constant : Constant  Value=true  OutDataTypeStr=boolean
  Parse Status Word : MATLAB Function  TreatAsAtomicUnit=on
  Terminator{,1..15} (16 alike) : Terminator
  aboveLimit : Logic  IconShape=distinctive  AllPortsSameDT=off  OutDataTypeStr=boolean
  alarm : Logic  IconShape=distinctive  AllPortsSameDT=off  OutDataTypeStr=boolean
  atSetpoint : Logic  IconShape=distinctive  AllPortsSameDT=off  OutDataTypeStr=boolean
  commErr : Logic  IconShape=distinctive  AllPortsSameDT=off  OutDataTypeStr=boolean
  extCtrlLoc : Logic  IconShape=distinctive  AllPortsSameDT=off  OutDataTypeStr=boolean
  extRunEnable : Logic  IconShape=distinctive  AllPortsSameDT=off  OutDataTypeStr=boolean
  mswB13 : Logic  IconShape=distinctive  AllPortsSameDT=off  OutDataTypeStr=boolean
  mswB14 : Logic  IconShape=distinctive  AllPortsSameDT=off  OutDataTypeStr=boolean
  off2 : Logic  IconShape=distinctive  AllPortsSameDT=off  OutDataTypeStr=boolean
  off3 : Logic  IconShape=distinctive  AllPortsSameDT=off  OutDataTypeStr=boolean
  rdyOn : Logic  IconShape=distinctive  AllPortsSameDT=off  OutDataTypeStr=boolean
  rdyRef : Logic  IconShape=distinctive  AllPortsSameDT=off  OutDataTypeStr=boolean
  rdyRun : Logic  IconShape=distinctive  AllPortsSameDT=off  OutDataTypeStr=boolean
  remote : Logic  IconShape=distinctive  AllPortsSameDT=off  OutDataTypeStr=boolean
  switchOnInhibit : Logic  IconShape=distinctive  AllPortsSameDT=off  OutDataTypeStr=boolean
  tripped : Logic  IconShape=distinctive  AllPortsSameDT=off  OutDataTypeStr=boolean
  wires:
  statusWord/1 -> Parse Status Word/1(StatusWord)
  Parse Status Word/1(rdy_on) -> rdyOn/2
  Constant/1 -> mswB13/1, commErr/1, mswB14/1, extRunEnable/1, extCtrlLoc/1, aboveLimit/1, remote/1, atSetpoint/1, alarm/1, switchOnInhibit/1, off3/1, off2/1, tripped/1, rdyRef/1, rdyRun/1, rdyOn/1
  rdyOn/1 -> Terminator/1
  rdyRun/1 -> Terminator1/1
  Parse Status Word/2(rdy_run) -> rdyRun/2
  rdyRef/1 -> Terminator2/1
  tripped/1 -> Terminator3/1
  Parse Status Word/4(tripped) -> tripped/2
  Parse Status Word/5(off2) -> off2/2
  off2/1 -> Terminator4/1
  off3/1 -> Terminator5/1
  Parse Status Word/6(off3) -> off3/2
  Parse Status Word/7(swc_on_inhib) -> switchOnInhibit/2
  switchOnInhibit/1 -> Terminator6/1
  alarm/1 -> Terminator7/1
  Parse Status Word/8(alarm) -> alarm/2
  Parse Status Word/9(at_setpoint) -> atSetpoint/2
  atSetpoint/1 -> Terminator8/1
  remote/1 -> Terminator9/1
  Parse Status Word/10(remote) -> remote/2
  Parse Status Word/11(above_limit) -> aboveLimit/2
  aboveLimit/1 -> Terminator10/1
  extCtrlLoc/1 -> Terminator11/1
  Parse Status Word/12(ext_ctrl_loc) -> extCtrlLoc/2
  Parse Status Word/13(ext_run_enable) -> extRunEnable/2
  extRunEnable/1 -> Terminator12/1
  mswB13/1 -> Terminator13/1
  Parse Status Word/14(msw_b13) -> mswB13/2
  Parse Status Word/15(msw_b14) -> mswB14/2
  mswB14/1 -> Terminator14/1
  commErr/1 -> Terminator15/1
  Parse Status Word/16(comm_err) -> commErr/2
  Parse Status Word/3(rdy_ref) -> rdyRef/2

== system windEmulatorStep4/fileAndUI/hptoSignalsUI/powerCalcs ==
  hptoSignals : Inport  OutDataTypeStr=Bus: hptoSignalBus
  Bus Selector : BusSelector  OutputSignals=pressure_bar,genPumpFlow_lpm
  Bus Selector1 : BusSelector  OutputSignals=excShaftSpeed_rpm,excShaftTorque_Nm
  Moving Average : dspstat3/Moving Average  Method=Sliding window  ForgettingFactorPort=off  SpecifyWindowLength=on  WindowLength=movingAverageLength  OverlapLength=2499  AllowArbitraryInputLength=off  ForgettingFactor=0.9  SimulateUsing=Code generation
  Moving Average1 : dspstat3/Moving Average  Method=Sliding window  ForgettingFactorPort=off  SpecifyWindowLength=on  WindowLength=movingAverageLength  OverlapLength=2499  AllowArbitraryInputLength=off  ForgettingFactor=0.9  SimulateUsing=Code generation
  Product : Product
  Product1 : Product
  Terminator{,1..3} (4 alike) : Terminator
  bar->Pa : Gain  Gain=bar2pa
  excShaftPowerAverage_W : Gain
  excShaftPower_W : Gain
  hydrPowerAverage_W : Gain
  hydrPower_W : Gain
  "l/m -> m3/s" : Gain  Gain=lpm2m3ps
  "rpm -> rad/s" : Gain  Gain=rpm2radps
  wires:
  hptoSignals/1 -> Bus Selector1/1, Bus Selector/1
  Bus Selector/1 -> bar->Pa/1  "<pressure_bar>"
  bar->Pa/1 -> Product/1
  Bus Selector/2 -> "l/m -> m3/s"/1  "<genPumpFlow_lpm>"
  "l/m -> m3/s"/1 -> Product/2
  Product/1 -> Moving Average/1, hydrPower_W/1
  hydrPower_W/1 -> Terminator/1
  Moving Average/1 -> hydrPowerAverage_W/1
  hydrPowerAverage_W/1 -> Terminator1/1
  Bus Selector1/1 -> "rpm -> rad/s"/1  "<excShaftSpeed_rpm>"
  "rpm -> rad/s"/1 -> Product1/1
  Bus Selector1/2 -> Product1/2  "<excShaftTorque_Nm>"
  excShaftPower_W/1 -> Terminator2/1
  Moving Average1/1 -> excShaftPowerAverage_W/1
  excShaftPowerAverage_W/1 -> Terminator3/1
  Product1/1 -> excShaftPower_W/1, Moving Average1/1

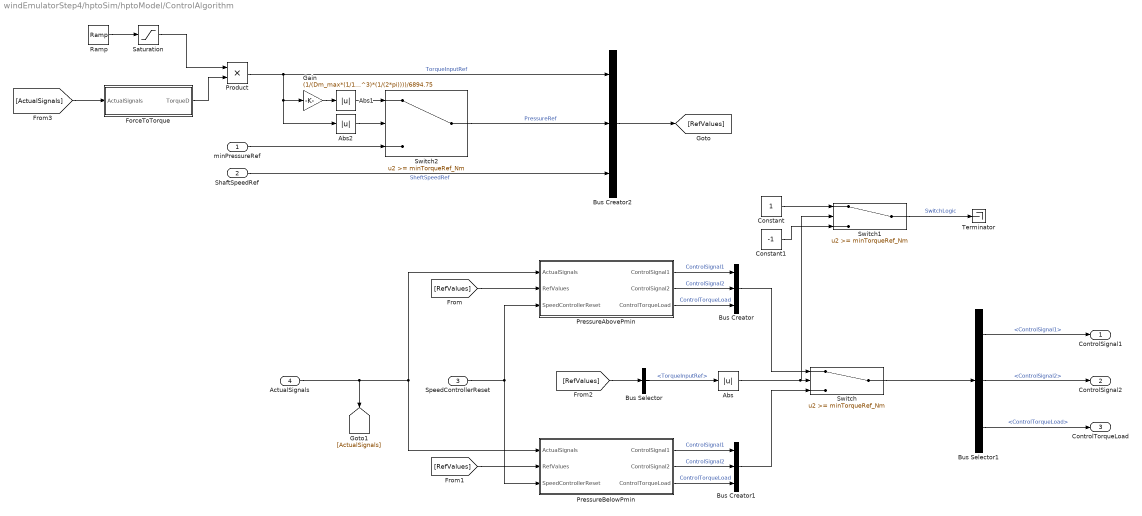
== system windEmulatorStep4/hptoSim/hptoModel/ControlAlgorithm ==
  minPressureRef : Inport
  ShaftSpeedRef : Inport  Port=2
  SpeedControllerReset : Inport  Port=3
  ActualSignals : Inport  Port=4
  Abs : Abs  SaturateOnIntegerOverflow=off
  Abs1 : Abs  SaturateOnIntegerOverflow=off
  Abs2 : Abs  SaturateOnIntegerOverflow=off
  Bus Creator : BusCreator  Inputs=3
  Bus Creator1 : BusCreator  Inputs=3
  Bus Creator2 : BusCreator  Inputs=3
  Bus Selector : BusSelector  OutputSignals=TorqueInputRef
  Bus Selector1 : BusSelector  OutputSignals=ControlSignal1,ControlSignal2,ControlTorqueLoad
  Constant : Constant
  Constant1 : Constant  Value=-1
  ForceToTorque : Subsystem
  Gain : Gain  Gain=(1/(Dm_max*(1/100^3)*(1/(2*pi))))/6894.75
  PressureAbovePmin : Subsystem
  PressureBelowPmin : Subsystem
  Product : Product
  Ramp : simulink/Sources/Ramp  slope=1/10  start=10  InitialOutput=0
  Saturation : Saturate  UpperLimit=1  LowerLimit=0
  Switch : Switch  Threshold=minTorqueRef_Nm  SaturateOnIntegerOverflow=off  InputSameDT=off
  Switch1 : Switch  Threshold=minTorqueRef_Nm  SaturateOnIntegerOverflow=off  InputSameDT=off
  Switch2 : Switch  Threshold=minTorqueRef_Nm  SaturateOnIntegerOverflow=off  InputSameDT=off
  Terminator : Terminator
  ControlSignal1 : Outport
  ControlSignal2 : Outport  Port=2
  ControlTorqueLoad : Outport  Port=3
  wires:
  ActualSignals/1 -> [ActualSignals], PressureAbovePmin/1(ActualSignals), PressureBelowPmin/1(ActualSignals)
  PressureAbovePmin/1(ControlSignal1) -> Bus Creator/1  "ControlSignal1"
  PressureAbovePmin/2(ControlSignal2) -> Bus Creator/2  "ControlSignal2"
  PressureAbovePmin/3(ControlTorqueLoad) -> Bus Creator/3  "ControlTorqueLoad"
  Bus Creator/1 -> Switch/1
  PressureBelowPmin/1(ControlSignal1) -> Bus Creator1/1  "ControlSignal1"
  PressureBelowPmin/2(ControlSignal2) -> Bus Creator1/2  "ControlSignal2"
  PressureBelowPmin/3(ControlTorqueLoad) -> Bus Creator1/3  "ControlTorqueLoad"
  Bus Creator1/1 -> Switch/3
  Bus Selector1/1 -> ControlSignal1/1  "<ControlSignal1>"
  Bus Selector1/2 -> ControlSignal2/1  "<ControlSignal2>"
  Bus Selector1/3 -> ControlTorqueLoad/1  "<ControlTorqueLoad>"
  Product/1 -> Bus Creator2/1, Abs2/1, Gain/1  "TorqueInputRef"
  ShaftSpeedRef/1 -> Bus Creator2/3  "SheftSpeedRef"
  Bus Creator2/1 -> [RefValues]
  [RefValues] -> PressureAbovePmin/2(RefValues)
  [RefValues] -> PressureBelowPmin/2(RefValues)
  [RefValues] -> Bus Selector/1
  Bus Selector/1 -> Abs/1  "<TorqueInputRef>"
  Abs/1 -> Switch1/2, Switch/2
  Constant/1 -> Switch1/1
  Constant1/1 -> Switch1/3
  Switch1/1 -> Terminator/1  "SwitchLogic"
  Gain/1 -> Abs1/1
  Abs1/1 -> Switch2/1
  minPressureRef/1 -> Switch2/3
  Abs2/1 -> Switch2/2
  Switch2/1 -> Bus Creator2/2  "PressureRef"
  Saturation/1 -> Product/1
  Ramp/1 -> Saturation/1
  [ActualSignals] -> ForceToTorque/1(ActualSignals)
  ForceToTorque/1(TorqueD) -> Product/2
  Switch/1 -> Bus Selector1/1
  SpeedControllerReset/1 -> PressureAbovePmin/3(SpeedControllerReset), PressureBelowPmin/3(SpeedControllerReset)
